simulink model "lab7"  (R2020b)
settings: Solver=VariableStepAuto  StartTime=0.0  StopTime=10.0  RelTol=1e-3
settings Model: Creator=karth  LastModifiedBy=karth

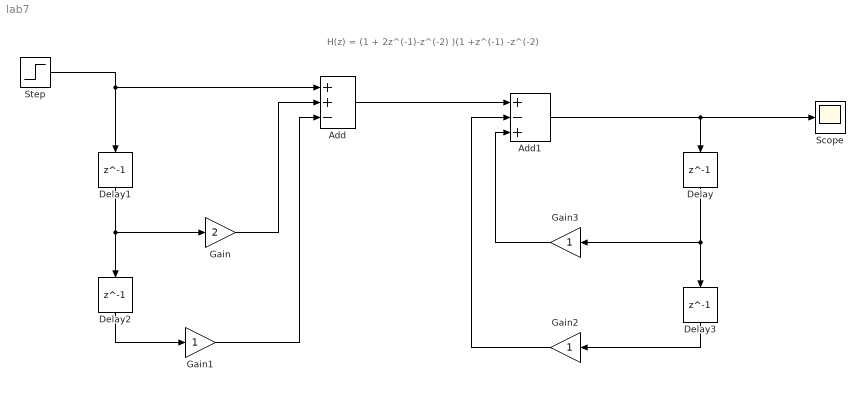
== system lab7 ==
  note: H(z) = (1 + 2z^(-1)-z^(-2) )(1 +z^(-1) -z^(-2)
  Add : Sum  Inputs=++-
  Add1 : Sum  Inputs=+-+
  Delay{,1..3} (4 alike) : Delay  DelayLength=1  InitialCondition=0
  Gain : Gain  Gain=2
  Gain1 : Gain
  Gain2 : Gain
  Gain3 : Gain
  Scope : Scope
  Step : Step  SampleTime=0
  wires:
  Delay1/1 -> Gain/1, Delay2/1
  Delay2/1 -> Gain1/1
  Step/1 -> Add/1, Delay1/1
  Gain/1 -> Add/2
  Gain1/1 -> Add/3
  Add/1 -> Add1/1
  Delay/1 -> Gain3/1, Delay3/1
  Add1/1 -> Delay/1, Scope/1
  Delay3/1 -> Gain2/1
  Gain3/1 -> Add1/3
  Gain2/1 -> Add1/2
